simulink model "Model_9"  (R2020b)
settings: Solver=VariableStepAuto  StartTime=0.0  StopTime=10.0  RelTol=1e-3
settings Model: Creator=Akarsh  LastModifiedBy=Akarsh

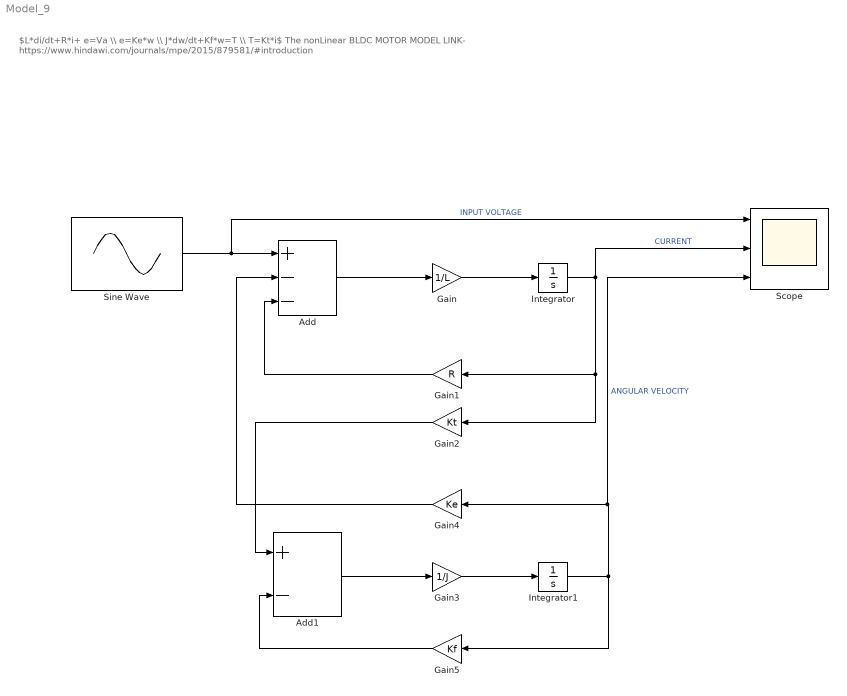
== system Model_9 ==
  note: $L*di/dt+R*i+ e=Va \\ e=Ke*w \\ J*dw/dt+Kf*w=T \\ T=Kt*i$
      | The nonLinear BLDC MOTOR MODEL
      | LINK- https://www.hindawi.com/journals/mpe/2015/879581/#introduction
  Add : Sum  Inputs=+--
  Add1 : Sum  Inputs=+-
  Gain : Gain  Gain=1/L  mask{L=0.003}
  Gain1 : Gain  Gain=R  mask{R=0.95}
  Gain2 : Gain  Gain=Kt  mask{Kt=0.5}
  Gain3 : Gain  Gain=1/J  mask{J=0.0008}
  Gain4 : Gain  Gain=Ke  mask{Ke=0.008}
  Gain5 : Gain  Gain=Kf  mask{Kf=0.003}
  Integrator : Integrator
  Integrator1 : Integrator
  Scope : Scope  NumInputPorts=3
  Sine Wave : Sin  SampleTime=0
  wires:
  Add/1 -> Gain/1
  Gain/1 -> Integrator/1
  Gain1/1 -> Add/3
  Integrator/1 -> Gain1/1, Gain2/1, Scope/2  "CURRENT"
  Gain2/1 -> Add1/1
  Add1/1 -> Gain3/1
  Gain3/1 -> Integrator1/1
  Integrator1/1 -> Scope/3, Gain4/1, Gain5/1  "ANGULAR VELOCITY"
  Gain4/1 -> Add/2
  Gain5/1 -> Add1/2
  Sine Wave/1 -> Add/1, Scope/1  "INPUT VOLTAGE"
